simulink model "LEGO_NXT_M1V4_Closed_Loop_DC_Motor_Position_Control"  (R2015a)
settings: Solver=FixedStepDiscrete  SolverMode=SingleTasking  StartTime=0.0  StopTime=inf  FixedStep=.03  RelTol=1e-3
libraries: MinSegLibrary_M1V4 x2
settings Model: SimulationMode=external  ExtModeTrigDuration=2  Creator=malcoj2  LastModifiedBy=hurstj
settings OptimizationCC: OptimizeModelRefInitCode=on  LifeSpan=1
settings DebuggingCC: UnderspecifiedInitializationDetection=Classic  MergeDetectMultiDrivingBlocksExec=none  StateNameClashWarn=warning
settings HardwareCC: ProdBitPerInt=16  ProdBitPerPointer=8  ProdIntDivRoundTo=Zero  ProdEndianess=LittleEndian  ProdWordSize=8  ProdHWDeviceType=Atmel->AVR
settings RTWCC: SystemTargetFile=realtime.tlc  GenerateMakefile=off  TemplateMakefile=realtime.tmf  Description=Run on Target Hardware  RTWVerbose=off
settings ERTTargetCC: CombineOutputUpdateFcns=off  ExtMode=on  ExtModeTransport=3  ExtModeMexArgs=0 71 115200  ERTSrcFileBannerTemplate=realtime_code_template.cgt  ERTHdrFileBannerTemplate=realtime_code_template.cgt  ERTDataSrcFileTemplate=realtime_code_template.cgt  ERTDataHdrFileTemplate=realtime_code_template.cgt  ERTCustomFileTemplate=realtime_file_process.tlc

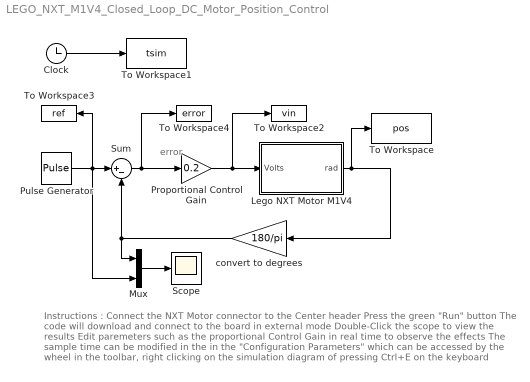
== system LEGO_NXT_M1V4_Closed_Loop_DC_Motor_Position_Control ==
  note: error
  note: Instructions :
      | Connect the NXT Motor connector to the Center header
      | Press the green "Run" button
      | The code will download and connect to the board in external mode
      | Double-Click the scope to view the results
      | Edit paremeters such as the proportional Control Gain in real time to observe the effects
      |
      | The sample time can be modified in the in the "Configuration Parameters" which can be accessed by the wheel in the toolbar, right clicking on the simulation diagram of pressing Ctrl+E on the keyboard
  Clock : Clock
  Lego NXT Motor M1V4 : Subsystem
  Mux : Mux  Inputs=2
  Proportional Control Gain : Gain  Gain=0.2
  Pulse Generator : DiscretePulseGenerator  PulseType=Time based  Amplitude=90  Period=3  PulseWidth=50
  Scope : Scope
      settings: TimeRange=15  YMin=-20  YMax=120
  Sum : Sum  Inputs=|+-
  To Workspace : ToWorkspace  VariableName=pos  SampleTime=-1
  To Workspace1 : ToWorkspace  VariableName=tsim  SampleTime=-1
  To Workspace2 : ToWorkspace  VariableName=vin  SampleTime=-1
  To Workspace3 : ToWorkspace  VariableName=ref  SampleTime=-1
  To Workspace4 : ToWorkspace  VariableName=error  SampleTime=-1
  convert to degrees : Gain  Gain=180/pi
  wires:
  Sum/1 -> Proportional Control Gain/1, To Workspace4/1
  Clock/1 -> To Workspace1/1
  Pulse Generator/1 -> Mux/2, To Workspace3/1, Sum/1
  convert to degrees/1 -> Mux/1, Sum/2
  Mux/1 -> Scope/1
  Lego NXT Motor M1V4/1(rad) -> convert to degrees/1, To Workspace/1
  Proportional Control Gain/1 -> Lego NXT Motor M1V4/1(Volts), To Workspace2/1

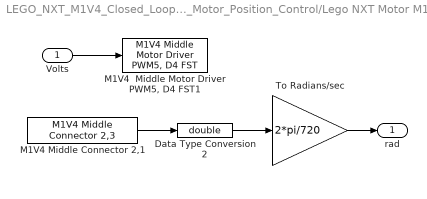
== system LEGO_NXT_M1V4_Closed_Loop_DC_Motor_Position_Control/Lego NXT Motor M1V4 ==
  Volts : Inport
  Data Type Conversion2 : DataTypeConversion  OutDataTypeStr=double
  "M1V4  Middle Motor Driver PWM5, D4 FST1" : MinSegLibrary_M1V4/M1V4  Middle Motor Driver PWM5, D4 FST  Vsupply=3.25
  M1V4 Middle Connector 2,1 : MinSegLibrary_M1V4/M1V4 Middle Connector 2,3  Encoder=0  PinA=3  PinB=2  PWMFSelect=3  PWMTimer=-1
  To Radians/sec : Gain  Gain=2*pi/720
  rad : Outport
  wires:
  To Radians/sec/1 -> rad/1
  M1V4 Middle Connector 2,1/1 -> Data Type Conversion2/1
  Volts/1 -> "M1V4  Middle Motor Driver PWM5, D4 FST1"/1
  Data Type Conversion2/1 -> To Radians/sec/1
